simulink model "controls_INDI"  (R2020a)
settings: Solver=FixedStepAuto  StartTime=0.0  StopTime=20  FixedStep=1/par.freq  RelTol=1e-3
undefined symbols (not defined in the file): INDI, INDI_DRF, par
libraries: eeGeneralControl x4, simulink x1
settings Model: Creator=Matthias  LastModifiedBy=xueruiwang
settings DataIOCC: SaveOutput=off  SaveTime=off  ReturnWorkspaceOutputs=off
settings DebuggingCC: ModelReferenceExtraNoncontSigs=warning  ArithmeticOperatorsInVariantConditions=warning
settings ModelReferenceCC: ModelReferenceNumInstancesAllowed=Single
settings SFSimCC: CustomCodeUndefinedFunction=UseInterfaceOnly
settings GRTTargetCC: CombineOutputUpdateFcns=off  MatFileLogging=off

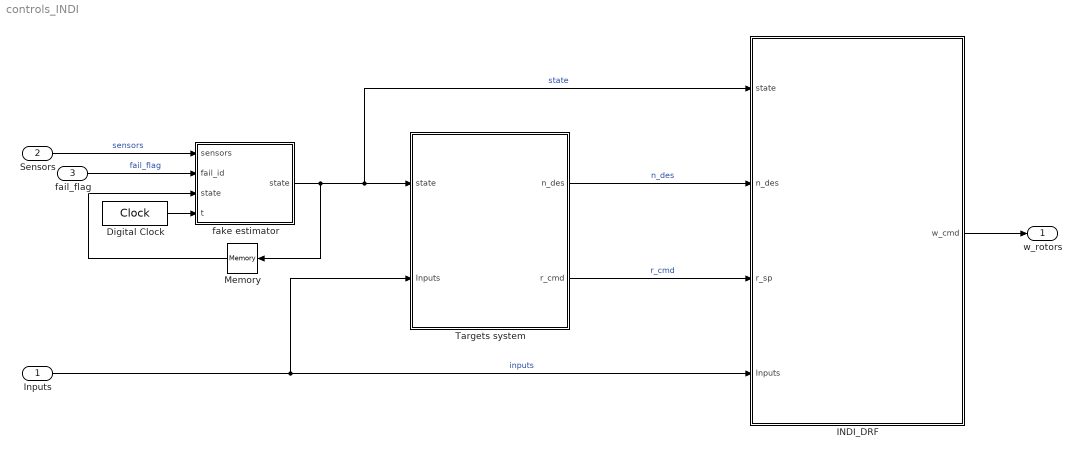
== system controls_INDI ==
  Inputs : Inport  OutDataTypeStr=Bus: inputsBus
  Sensors : Inport  Port=2  OutDataTypeStr=Bus: sensorsBus
  fail_flag : Inport  Port=3  OutDataTypeStr=double  PortDimensions=1
  Digital Clock : DigitalClock  SampleTime=1/par.freq
  INDI_DRF : Subsystem  AncestorBlock=INDI/INDI_DRF
  Memory : Memory
  Targets system : Subsystem
  "fake estimator " : MATLAB Function  TreatAsAtomicUnit=on
  w_rotors : Outport  VectorParamsAs1DForOutWhenUnconnected=off
  wires:
  fail_flag/1 -> "fake estimator "/2(fail_id)  "fail_flag"
  Targets system/2(r_cmd) -> INDI_DRF/3(r_sp)  "r_cmd"
  "fake estimator "/1(state) -> Memory/1, INDI_DRF/1(state), Targets system/1(state)  "state"
  Inputs/1 -> Targets system/2(Inputs), INDI_DRF/4(Inputs)  "inputs"
  INDI_DRF/1(w_cmd) -> w_rotors/1
  Targets system/1(n_des) -> INDI_DRF/2(n_des)  "n_des"
  Sensors/1 -> "fake estimator "/1(sensors)  "sensors"
  Memory/1 -> "fake estimator "/3("state ")
  Digital Clock/1 -> "fake estimator "/4(t)

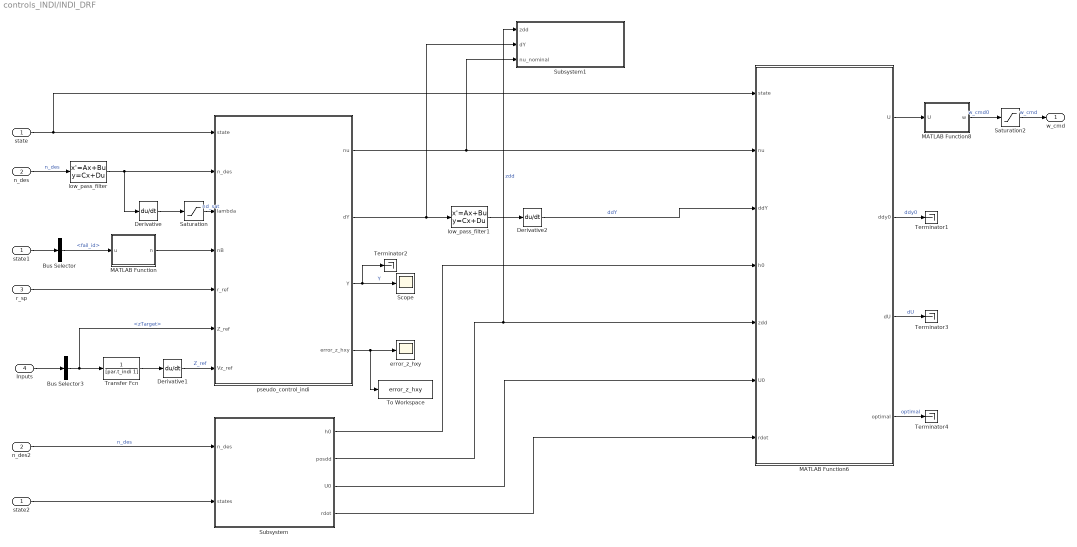
== system controls_INDI/INDI_DRF ==
  state : Inport
  n_des : Inport  Port=2  PortDimensions=3
  r_sp : Inport  Port=3
  Inputs : Inport  Port=4
  Bus Selector : BusSelector  OutputSignals=fail_id
  Bus Selector3 : BusSelector  OutputSignals=zTarget
  Derivative : Derivative
  Derivative1 : Derivative
  Derivative2 : Derivative
  MATLAB Function : MATLAB Function  TreatAsAtomicUnit=on
  MATLAB Function6 : MATLAB Function  TreatAsAtomicUnit=on
  MATLAB Function8 : MATLAB Function  TreatAsAtomicUnit=on
  Saturation : Saturate
  Saturation2 : Saturate  UpperLimit=par.w_max  LowerLimit=par.w_min
  Scope : Scope
  Subsystem : Subsystem
  Subsystem1 : Subsystem
  Terminator{1..4} (4 alike) : Terminator
  To Workspace : ToWorkspace  VariableName=error_z_hxy  SampleTime=-1
      settings: Save2DSignal=2-D array (concatenate along first dimension)
  Transfer Fcn : TransferFcn  Denominator=[par.t_indi 1]
  error_z_hxy : Scope
  low_pass_filter : StateSpace  A=-diag([1/par.t_indi, 1/par.t_indi, 1/par.t_indi])  B=diag([1/par.t_indi, 1/par.t_indi, 1/par.t_indi])  C=eye(3)  D=zeros(3,3)  InitialCondition=[0,0,-1]
  low_pass_filter1 : StateSpace  A=-diag([1/par.t_indi, 1/par.t_indi])  B=diag([1/par.t_indi, 1/par.t_indi])  C=eye(2)  D=zeros(2,2)  InitialCondition=0
  n_des2 : InportShadow  Port=2  PortDimensions=3
  pseudo_control_indi : MATLAB Function  TreatAsAtomicUnit=on
  state1 : InportShadow
  state2 : InportShadow
  w_cmd : Outport  VectorParamsAs1DForOutWhenUnconnected=off
  wires:
  MATLAB Function6/1(U) -> MATLAB Function8/1(U)
  pseudo_control_indi/3(Y) -> Terminator2/1, Scope/1  "Y"
  Saturation/1 -> pseudo_control_indi/3(lambda)  "nd_sat"
  Derivative/1 -> Saturation/1
  low_pass_filter/1 -> Derivative/1, pseudo_control_indi/2(n_des)
  MATLAB Function6/2(ddy0) -> Terminator1/1  "ddy0"
  state1/1 -> Bus Selector/1
  state/1 -> pseudo_control_indi/1(state), MATLAB Function6/1(state)
  state2/1 -> Subsystem/2(states)
  Bus Selector/1 -> MATLAB Function/1(u)  "<fail_id>"
  Subsystem/4(rdot) -> MATLAB Function6/7(rdot)
  Subsystem/3(U0) -> MATLAB Function6/6(U0)
  Subsystem/2(posdd) -> MATLAB Function6/5(zdd), Subsystem1/1(zdd)  "zdd"
  Subsystem/1(h0) -> MATLAB Function6/4(h0)
  n_des2/1 -> Subsystem/1(n_des)  "n_des"
  low_pass_filter1/1 -> Derivative2/1
  Derivative2/1 -> MATLAB Function6/3(ddY)  "ddY"
  pseudo_control_indi/2(dY) -> Subsystem1/2(dY), low_pass_filter1/1
  Saturation2/1 -> w_cmd/1  "w_cmd"
  n_des/1 -> low_pass_filter/1  "n_des"
  MATLAB Function8/1(w) -> Saturation2/1  "w_cmd0"
  MATLAB Function/1(n) -> pseudo_control_indi/4(nB)
  Transfer Fcn/1 -> Derivative1/1
  Bus Selector3/1 -> Transfer Fcn/1, pseudo_control_indi/6(Z_ref)  "<zTarget>"
  Derivative1/1 -> pseudo_control_indi/7(Vz_ref)  "Z_ref"
  r_sp/1 -> pseudo_control_indi/5(r_ref)
  Inputs/1 -> Bus Selector3/1
  MATLAB Function6/3(dU) -> Terminator3/1  "dU"
  MATLAB Function6/4(optimal) -> Terminator4/1  "optimal"
  pseudo_control_indi/4(error_z_hxy) -> To Workspace/1, error_z_hxy/1
  pseudo_control_indi/1(nu) -> Subsystem1/3(nu_nominal), MATLAB Function6/2(nu)

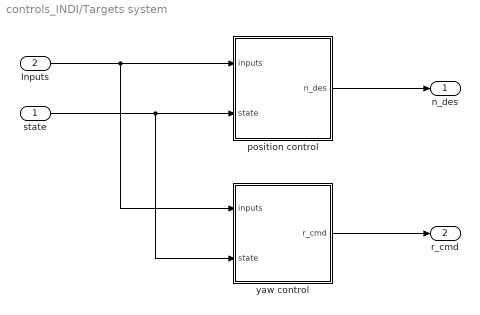
== system controls_INDI/Targets system ==
  state : Inport
  Inputs : Inport  Port=2
  position control : MATLAB Function  TreatAsAtomicUnit=on
  yaw control : MATLAB Function  TreatAsAtomicUnit=on
  n_des : Outport  VectorParamsAs1DForOutWhenUnconnected=off
  r_cmd : Outport  Port=2  VectorParamsAs1DForOutWhenUnconnected=off
  wires:
  yaw control/1(r_cmd) -> r_cmd/1
  Inputs/1 -> yaw control/1(inputs), position control/1(inputs)
  state/1 -> yaw control/2(state), position control/2(state)
  position control/1(n_des) -> n_des/1

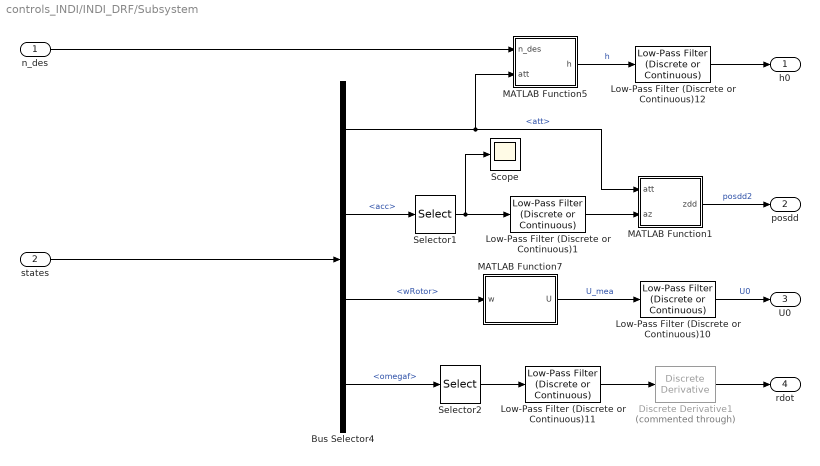
== system controls_INDI/INDI_DRF/Subsystem ==
  n_des : Inport
  states : Inport  Port=2
  Bus Selector4 : BusSelector  OutputSignals=att,acc,wRotor,omegaf
  Discrete Derivative1 : simulink/Discrete/Discrete Derivative  Commented=through  gainval=1.0  ICPrevScaledInput=0.0  OutMin=[]  OutMax=[]  OutDataType=fixdt(1, 16)  OutScaling=2^-10  DoSatur=off
  Low-Pass Filter (Discrete or Continuous){1,10..12} (4 alike) : eeGeneralControl/Low-Pass Filter (Discrete or Continuous)  K=1  T=par.t_indi  B=inf  A=-inf  init_option=Inherited from block input  x0=0  Ts=-1
  MATLAB Function1 : MATLAB Function  TreatAsAtomicUnit=on
  MATLAB Function5 : MATLAB Function  TreatAsAtomicUnit=on
  MATLAB Function7 : MATLAB Function  TreatAsAtomicUnit=on
  Scope : Scope
  Selector1 : Selector  InputPortWidth=3  IndexOptions=Index vector (dialog)  Indices=3  OutputSizes=1
  Selector2 : Selector  InputPortWidth=3  IndexOptions=Index vector (dialog)  Indices=3  OutputSizes=1
  h0 : Outport  VectorParamsAs1DForOutWhenUnconnected=off
  posdd : Outport  Port=2  VectorParamsAs1DForOutWhenUnconnected=off
  U0 : Outport  Port=3  VectorParamsAs1DForOutWhenUnconnected=off
  rdot : Outport  Port=4  VectorParamsAs1DForOutWhenUnconnected=off
  wires:
  MATLAB Function1/1(zdd) -> posdd/1  "posdd2"
  Low-Pass Filter (Discrete or Continuous)1/1 -> MATLAB Function1/2(az)
  Bus Selector4/2 -> Selector1/1  "<acc>"
  n_des/1 -> MATLAB Function5/1(n_des)
  Low-Pass Filter (Discrete or Continuous)12/1 -> h0/1
  Low-Pass Filter (Discrete or Continuous)11/1 -> Discrete Derivative1/1
  Low-Pass Filter (Discrete or Continuous)10/1 -> U0/1  "U0"
  MATLAB Function7/1(U) -> Low-Pass Filter (Discrete or Continuous)10/1  "U_mea"
  Selector2/1 -> Low-Pass Filter (Discrete or Continuous)11/1
  MATLAB Function5/1(h) -> Low-Pass Filter (Discrete or Continuous)12/1  "h"
  states/1 -> Bus Selector4/1
  Bus Selector4/1 -> MATLAB Function1/1(att), MATLAB Function5/2(att)  "<att>"
  Bus Selector4/3 -> MATLAB Function7/1(w)  "<wRotor>"
  Bus Selector4/4 -> Selector2/1  "<omegaf>"
  Discrete Derivative1/1 -> rdot/1
  Selector1/1 -> Scope/1, Low-Pass Filter (Discrete or Continuous)1/1

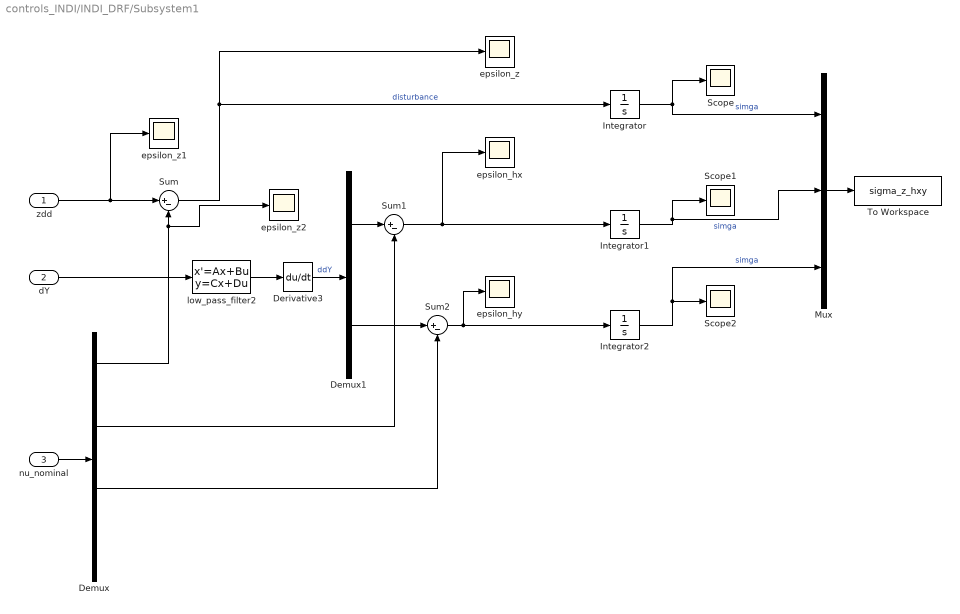
== system controls_INDI/INDI_DRF/Subsystem1 ==
  zdd : Inport
  dY : Inport  Port=2
  nu_nominal : Inport  Port=3
  Demux : Demux
  Demux1 : Demux  Outputs=2
  Derivative3 : Derivative
  Integrator : Integrator
  Integrator1 : Integrator
  Integrator2 : Integrator
  Mux : Mux  Inputs=3
  Scope : Scope
  Scope1 : Scope
  Scope2 : Scope
  Sum : Sum  Inputs=|+-
  Sum1 : Sum  Inputs=|+-
  Sum2 : Sum  Inputs=|+-
  To Workspace : ToWorkspace  VariableName=sigma_z_hxy  SampleTime=-1
      settings: Save2DSignal=2-D array (concatenate along first dimension)
  epsilon_hx : Scope
  epsilon_hy : Scope
  epsilon_z : Scope
  epsilon_z1 : Scope
  epsilon_z2 : Scope
  low_pass_filter2 : StateSpace  A=-diag([1/par.t_smdo, 1/par.t_smdo])  B=diag([1/par.t_smdo, 1/par.t_smdo])  C=eye(2)  D=zeros(2,2)  InitialCondition=0
  wires:
  low_pass_filter2/1 -> Derivative3/1
  nu_nominal/1 -> Demux/1
  zdd/1 -> epsilon_z1/1, Sum/1
  dY/1 -> low_pass_filter2/1
  Derivative3/1 -> Demux1/1  "ddY"
  Demux1/1 -> Sum1/1
  Demux1/2 -> Sum2/1
  Sum1/1 -> epsilon_hx/1, Integrator1/1
  Sum2/1 -> Integrator2/1, epsilon_hy/1
  Demux/3 -> Sum2/2
  Demux/2 -> Sum1/2
  Demux/1 -> epsilon_z2/1, Sum/2
  Sum/1 -> Integrator/1, epsilon_z/1  "disturbance"
  Integrator/1 -> Scope/1, Mux/1  "simga"
  Integrator1/1 -> Mux/2, Scope1/1  "simga"
  Integrator2/1 -> Mux/3, Scope2/1  "simga"
  Mux/1 -> To Workspace/1

== matlab function controls_INDI/INDI_DRF/Subsystem/MATLAB Function7 ==
  data: w input; U output
function U = omega2U(w)
%#codegen

U = zeros(4,1);
U(1) = w(1)^2;
U(2) = w(2)^2;
U(3) = w(3)^2;
U(4) = w(4)^2;
end

== matlab function controls_INDI/INDI_DRF/pseudo_control_indi ==
  data: state input; n_des input; lambda input; nB input; r_ref input; Z_ref input; Vz_ref input; nu output; par parameter; dY output; Y output; error_z_hxy output
function [nu,dY, Y,error_z_hxy] = pseudo_control_att_indi(state, n_des, lambda, nB, r_ref, Z_ref, Vz_ref, par)

[nu, dY, Y,error_z_hxy] = pseudo_control_att_indi(state, n_des, lambda, nB, r_ref, Z_ref, Vz_ref, par);

end

== matlab function controls_INDI/INDI_DRF/MATLAB Function ==
  data: u input; n output; par parameter
function n = fcn(u,par)

a = par.axis_tilt;

if par.DRF_enable == 0 || par.DRF_enable == 1 
    if u == 1
       n = [-a, a, -1];   
    elseif u == 2
       n = [-a, -a, -1];
    elseif u == 3
       n = [a, -a, -1];
    elseif u == 4
       n = [a, a, -1];
    else
       n = [0, 0, -1];    
    end
else
   n = [0, 0, -1];
end

== matlab function controls_INDI/Targets system/position control ==
  settings: updateMethod=DISCRETE
  data: inputs input Bus: inputsBus; n_des output size=[1 3]; state input Bus: stateBus; par parameter
function n_des   = positionControl(inputs, state, par)

[n_des] = URpositionControl(inputs, state, par);

end

== matlab function controls_INDI/Targets system/yaw control ==
  data: inputs input Bus: inputsBus; r_cmd output; state input Bus: stateBus; par parameter
function r_cmd = yawControl(inputs, state, par)

[r_cmd] = URYawControl(inputs, state, par);

end

== matlab function controls_INDI/fake estimator  ==
  data: sensors input; fail_id input; state input Bus: stateBus; state output; t input
function state  = fcn(sensors, fail_id, state,t)

state = UREstimators(sensors, fail_id, state,t);

end

== matlab function controls_INDI/INDI_DRF/MATLAB Function6 ==
  settings: updateMethod=DISCRETE
  data: state input; nu input; ddY input; h0 input; zdd input; U0 input; rdot input; U output; par parameter; ddy0 output; dU output; optimal output
function [U,ddy0,dU, optimal]  =  allocation_att_indi(state, nu, ddY, h0, zdd, U0, rdot, par)

ddy0 = zeros(4,2);
if par.allocType == 1
    [U,ddy0(:,1),dU]  =  allocation_att_indi(state, nu, ddY, h0, zdd, U0, rdot, par);
    optimal = [1 0];
elseif par.allocType == 2
    [U,ddy0, dU, optimal]  =  allocation_qpindi(state, nu, ddY, h0, zdd, U0, rdot, par);
else
    error('invalide allocation method');
end
end

== matlab function controls_INDI/INDI_DRF/Subsystem/MATLAB Function1 ==
  data: att input; az input; zdd output
function zdd = fcn(att,az)

phi = att(1);
theta = att(2);

zdd = az*cos(theta)*cos(phi) + 9.8124;

== matlab function controls_INDI/INDI_DRF/MATLAB Function8 ==
  data: U input; w output
function w = U2omega(U)
%#codegen

w = zeros(4,1);
w(1) = sqrt(abs(U(1)))*sign(U(1));
w(2) = sqrt(abs(U(2)))*sign(U(2));
w(3) = sqrt(abs(U(3)))*sign(U(3));
w(4) = sqrt(abs(U(4)))*sign(U(4));

end

== matlab function controls_INDI/INDI_DRF/Subsystem/MATLAB Function5 ==
  data: n_des input; att input; h output
function h = fcn(n_des, att)

phi = att(1);
theta = att(2);
psi = att(3);

R_IB = euler2Rot(phi,theta,psi);

h = R_IB \ n_des;
